simulink model "regtemppid"  (R2025a)
settings: Solver=ode45  StartTime=0.0  StopTime=160000  FixedStep=0.1  RelTol=1e-3  EnableMultiTasking=on
PreLoadFcn:
  | variables;
InitFcn:
  | variables;
values from neighbouring files (symbols this model uses):
  demi_serie = 'A'    [variables.m]
  Kp = 1.05    [variables.m]
  serie = 6    [variables.m]
  set_up = 1    [variables.m]
  T1p = 139.41    [variables.m]
  T2p = 14.29    [variables.m]
  thetap = 9.07    [variables.m]
  Ts = 1    [variables.m]
libraries: simulink x1
settings Model: PacingRate=20  ExtModeTrigMode=oneshot  ExtModeArmWhenConnect=off  Creator=auto2  LastModifiedBy=sabir
settings SolverCC: AlgebraicLoopSolver=TrustRegion
settings DataIOCC: SaveFormat=Array  SignalLoggingSaveFormat=ModelDataLogs  SaveOutput=off  SaveTime=off  ReturnWorkspaceOutputs=off  SignalLoggingName=sigsOut
settings OptimizationCC: BooleanDataType=off  ExpressionDepthLimit=2147483647.0  InitFltsAndDblsToZero=on  LifeSpan=inf
settings DebuggingCC: SaveWithParameterizedLinksMsg=none  UnderspecifiedInitializationDetection=Classic  MergeDetectMultiDrivingBlocksExec=none  SignalResolutionControl=TryResolveAllWithWarning  MultiTaskDSMMsg=warning  MultiTaskCondExecSysMsg=none  FcnCallInpInsideContextMsg=warning  UnconnectedInputMsg=warning  UnconnectedOutputMsg=warning  UnconnectedLineMsg=warning  StateNameClashWarn=warning  SFUnexpectedBacktrackingDiag=warning  SFNoUnconditionalDefaultTransitionDiag=warning  SFExecutionAtInitializationDiag=none  ArithmeticOperatorsInVariantConditions=warning
settings HardwareCC: ProdBitPerPointer=32.0  ProdBitPerSizeT=32.0  ProdBitPerPtrDiffT=32.0  ProdLargestAtomicFloat=None  ProdIntDivRoundTo=Undefined  ProdEndianess=Unspecified  ProdWordSize=32.0  ProdHWDeviceType=32-bit Generic  TargetUnknown=on
settings ModelReferenceCC: EnableRefExpFcnMdlSchedulingChecks=on  PropagateSignalLabelsOutOfModel=off
settings SFSimCC: SimUseLocalCustomCode=off  CustomCodeUndefinedFunction=UseInterfaceOnly
settings RTWCC: RTWUseLocalCustomCode=off  GPUComputeCapability=3.5
settings CodeAppCC: StateflowObjectComments=on
settings GRTTargetCC: TargetLangStandard=C89/C90 (ANSI)  CombineOutputUpdateFcns=off  GRTInterface=on
settings ConfigComp: CovMetricSettings=dw  CovSaveCumulativeToWorkspaceVar=on  CovSaveSingleToWorkspaceVar=on  CovExternalEMLEnable=off  CovSFcnEnable=off

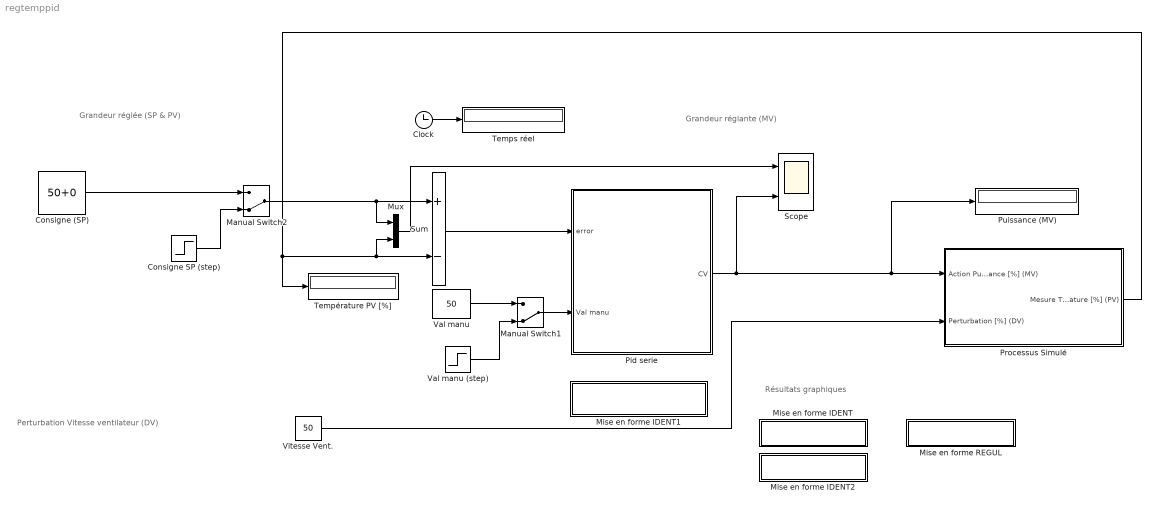
== system regtemppid ==
  note: Grandeur réglante (MV)
  note: Grandeur réglée (SP & PV)
  note: Perturbation Vitesse ventilateur (DV)
  note: Résultats graphiques
  Clock : Clock
      settings: StartFcn=simu(1).bloc_clock='labo'
  Consigne (SP) : Constant  StartFcn=simu(1,1).bloc_SP='labo'  Value=50+0
  Consigne SP (step) : Step  StartFcn=simu(1).bloc_Step_SP='labo'  Time=700  Before=45  After=55  SampleTime=0
  Manual Switch1 : ManualSwitch  CurrentSetting=0
  Manual Switch2 : ManualSwitch  CurrentSetting=0
  Mise en forme IDENT : Subsystem
      settings: OpenFcn=|
      | t=Scope_PID.time;A=[Scope_PID.signals.values];
      | y=A(:,2);u=A(:,3);
      | subplot(211)
      | plot(t,u,'black');
      | title('MV [%]')
      | subplot(212)
      | plot(t,y,'black');
      | title('PV [%]')
      | grid;figure(gcf)
      | 
      | 
      | 
      | tstep=find(diff(u)~=0);
      | tstep=tstep(end); % take last change
      | 
      | tm=t(tstep:end);
      | tm=tm-t(tstep);
      | um=u(tstep:end);
      | um=um-um(1);
      | ym=y(tstep:end);
      | ym=ym-ym(1);
      | 
      | y0 = y(tstep);
      | du = u(end)-u(tstep);
      mask Display: disp('Mise en forme IDENT')
  Mise en forme IDENT1 : Subsystem
      settings: OpenFcn=|
      | string_PID = get_param(bdroot, 'Name');
      | 
      | AMbit=3-length(get_param([string_PID '/Pid serie'],'AMbit'));
      | 
      | if AMbit==1,
      | set_param([string_PID '/Pid serie'],'AMbit','off');
      | AMbit=0;
      | elseif AMbit==0,
      | set_param([string_PID '/Pid serie'],'AMbit','on');
      | AMbit=1;
      | end
      | 
      | 
      | if AMbit==1,
      | 	set_param([string_PID '/Pid serie'],'BackgroundColor','red');
      | 	set_param([string_PID '/Pid serie'],'MaskDisplay','disp(''  PID \n [AUTO]'')');
      | end
      | if AMbit==0,
      | 	set_param([string_PID '/Pid serie'],'BackgroundColor','lightblue');
      | 	set_param([string_PID '/Pid serie'],'MaskDisplay','disp(''  PID \n [MANU]'')');
      | end
      mask Display: disp('Manu <->Auto')
  Mise en forme IDENT2 : Subsystem
      settings: OpenFcn=idoptregtemppidvdg;
      mask Display: disp('IDENT OPT VDG')
  Mise en forme REGUL : Subsystem
      settings: OpenFcn=|
      | t=Scope_PID.time;
      | A=[Scope_PID.signals.values];
      | ysp=A(:,1);
      | u=A(:,3);
      | y=A(:,2);
      | index=min(find(diff(ysp)))-99;
      | subplot(211);
      | y=y(index:end);
      | ysp=ysp(index:end);
      | t=t(index:end);
      | u=u(index:end);
      | plot(t,y,'black',t,ysp,'black');
      | grid;
      | title('PV [%] et SP [%]');
      | subplot(212),
      | plot(t,u,'black');
      | grid;
      | figure(gcf);
      | title('MV [%]')
      mask Display: disp('Mise en forme REGUL');
  Mux : Mux  Inputs=2
  Pid serie : Subsystem  StartFcn=simu(1).bloc_PID='labo'  mask{k=4.82, ti=168, td=10, tf=1, X0=50, lh=100, ll=0, AMbit=on}
      mask prompts: k "Gain"; ti "Temps d'intégration"; td "Temps de dérivation"; tf "Temps de filtrage"; X0 "Valeur initiale de la sortie"; lh "Limite Haute"; ll "Limite basse"; AMbit "Auto [v] / Manu [ ]"
      mask init:
      | string_PID = get_param(bdroot, 'Name');
      | 
      | AMbit=3-length(get_param([string_PID '/Pid serie'],'AMbit'));
      | if AMbit==1,
      | 	set_param([string_PID '/Pid serie'],'BackgroundColor','red');
      | 	set_param([string_PID '/Pid serie'],'MaskDisplay','disp(''  PID \n [AUTO]'')');
      | end
      | if AMbit==0, 
      | 	set_param([string_PID '/Pid serie'],'BackgroundColor','lightblue');
      | 	set_param([string_PID '/Pid serie'],'MaskDisplay','disp(''  PID \n [MANU]'')');
      | end
      mask Display: disp('  PID \n [AUTO]')
  Processus Simulé : Subsystem  StartFcn=simu(1).bloc_Process='labo'  mask{set_up=set_up, serie=serie, demi_serie=demi_serie}
      mask prompts: serie "Série"; demi_serie "Demi série"
      mask init:
      | %%%%%%%%%%%%%%%%%%%%%%%%%%%%%%%%%
      | 
      | switch set_up
      |    case 1
      |         Kd = -0.64;
      |         T1d = 81.54;
      |         T2d = 18.9;
      |         thetad = 12.49;
      |    case 2
      |         Kd = -0.43;
      |         T1d = 34.66;
      |         T2d = 1.13;
      |         thetad = 6.08; 
      |     case 3
      |         Kd = -0.34;
      |         T1d = 82.52;
      |         T2d = 20.99;
      |         thetad = 8.42;  
      | end
      | 
      | if (demi_serie == 'A')
      |     dserie = 1;
      | else
      |     dserie = 5;
      | end    
      | 
      | seed = str2num([num2str(serie) num2str(serie) num2str(dserie) num2str(set_up)]);
      | 
      | rng(seed)
      | x1 = (rand - 1)/5;
      | rng(seed+1)
      | x2 = (rand - 1)/5;
      | rng(seed+2)
      | x3 = (rand - 1)/5;
      | rng(seed+3)
      | x4 = (rand - 1)/5;
      | 
      | Kd = Kd*(1+x1);
      | T1d = T1d*(1+x2);
      | T2d = T2d*(1+x3);
      | thetad =thetad*(1+x4);
  Puissance (MV) : Display
      settings: StartFcn=simu(1).bloc_display_MV='labo'
  Scope : Scope  NumInputPorts=2
      settings: StartFcn=simu(1).bloc_display_scope='labo'  SampleTime=Ts  TimeSpan=1600  Title=SP [%] et PV [%]  ActiveDisplayYMinimum=-7.94952  ActiveDisplayYMaximum=71.54565  DataLoggingMaxPoints=25000  DataLoggingVariableName=Scope_PID
  Sum : Sum  Inputs=+-  InputSameDT=on  SaturateOnIntegerOverflow=on  OutDataTypeStr=Inherit: Same as first input
  Temps réel : Display
      settings: StartFcn=simu(1).bloc_display_clock='labo'
  Température PV [%] : Display
      settings: StartFcn=simu(1).bloc_Display_PV='labo'
  Val manu : Constant  StartFcn=simu(1).bloc_MV='labo'  Value=50
  Val manu (step) : Step  StartFcn=simu(1).bloc_Step_MV='labo'  Time=700  Before=50  After=60  SampleTime=0
  Vitesse Vent. : Constant  StartFcn=simu(1).bloc_DV='labo'  Value=50
  wires:
  Processus Simulé/1(Mesure Température [%] (PV)) -> Température PV [%]/1, Sum/2, Mux/2
  Manual Switch2/1 -> Sum/1, Mux/1
  Sum/1 -> Pid serie/1(error)
  Pid serie/1(CV) -> Processus Simulé/1(Action Puissance [%] (MV)), Puissance (MV)/1, Scope/2
  Vitesse Vent./1 -> Processus Simulé/2(Perturbation [%] (DV))
  Mux/1 -> Scope/1
  Clock/1 -> Temps réel/1
  Val manu (step)/1 -> Manual Switch1/2
  Val manu/1 -> Manual Switch1/1
  Manual Switch1/1 -> Pid serie/2(Val manu)
  Consigne SP (step)/1 -> Manual Switch2/2
  Consigne (SP)/1 -> Manual Switch2/1

== system regtemppid/Mise en forme IDENT ==

== system regtemppid/Mise en forme IDENT1 ==

== system regtemppid/Mise en forme IDENT2 ==

== system regtemppid/Mise en forme REGUL ==

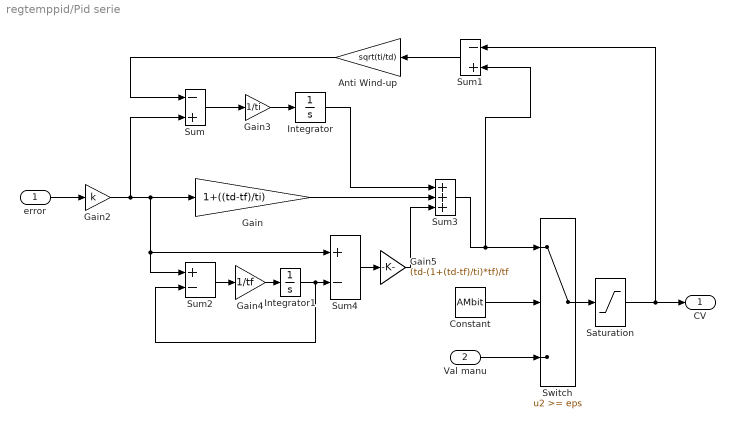
== system regtemppid/Pid serie ==
  error : Inport
  Val manu : Inport  Port=2
  Anti Wind-up : Gain  Gain=sqrt(ti/td)  SaturateOnIntegerOverflow=on  OutDataTypeStr=Inherit: Same as input  ParamDataTypeStr=Inherit: Same as input
  Constant : Constant  Value=AMbit
  Gain : Gain  Gain=1+((td-tf)/ti)  SaturateOnIntegerOverflow=on  OutDataTypeStr=Inherit: Same as input  ParamDataTypeStr=Inherit: Same as input
  Gain2 : Gain  Gain=k  SaturateOnIntegerOverflow=on  OutDataTypeStr=Inherit: Same as input  ParamDataTypeStr=Inherit: Same as input
  Gain3 : Gain  Gain=1/ti  SaturateOnIntegerOverflow=on  OutDataTypeStr=Inherit: Same as input  ParamDataTypeStr=Inherit: Same as input
  Gain4 : Gain  Gain=1/tf  SaturateOnIntegerOverflow=on  OutDataTypeStr=Inherit: Same as input  ParamDataTypeStr=Inherit: Same as input
  Gain5 : Gain  Gain=(td-(1+(td-tf)/ti)*tf)/tf  SaturateOnIntegerOverflow=on  OutDataTypeStr=Inherit: Same as input  ParamDataTypeStr=Inherit: Same as input
  Integrator : Integrator  InitialCondition=X0
  Integrator1 : Integrator
  Saturation : Saturate  UpperLimit=lh  LowerLimit=ll
  Sum : Sum  Inputs=-+  InputSameDT=on  SaturateOnIntegerOverflow=on  OutDataTypeStr=Inherit: Same as first input
  Sum1 : Sum  Inputs=-+  InputSameDT=on  SaturateOnIntegerOverflow=on  OutDataTypeStr=Inherit: Same as first input
  Sum2 : Sum  Inputs=+-  InputSameDT=on  SaturateOnIntegerOverflow=on  OutDataTypeStr=Inherit: Same as first input
  Sum3 : Sum  Inputs=+++  InputSameDT=on  SaturateOnIntegerOverflow=on  OutDataTypeStr=Inherit: Same as first input
  Sum4 : Sum  Inputs=+-  InputSameDT=on  SaturateOnIntegerOverflow=on  OutDataTypeStr=Inherit: Same as first input
  Switch : Switch  Threshold=eps
  CV : Outport
  wires:
  Saturation/1 -> Sum1/1, CV/1
  Switch/1 -> Saturation/1
  Val manu/1 -> Switch/3
  Constant/1 -> Switch/2
  error/1 -> Gain2/1
  Sum1/1 -> Anti Wind-up/1
  Anti Wind-up/1 -> Sum/1
  Sum3/1 -> Switch/1, Sum1/2
  Sum/1 -> Gain3/1
  Gain2/1 -> Sum/2, Gain/1, Sum2/1, Sum4/1
  Gain/1 -> Sum3/2
  Gain3/1 -> Integrator/1
  Integrator/1 -> Sum3/1
  Sum2/1 -> Gain4/1
  Gain4/1 -> Integrator1/1
  Sum4/1 -> Gain5/1
  Integrator1/1 -> Sum4/2, Sum2/2
  Gain5/1 -> Sum3/3

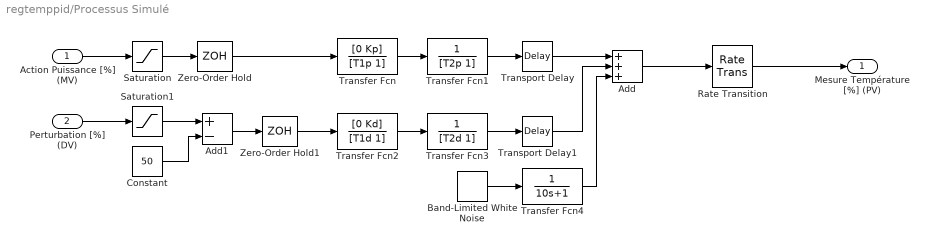
== system regtemppid/Processus Simulé ==
  Action Puissance [%] (MV) : Inport
  Perturbation [%] (DV) : Inport  Port=2
  Add : Sum  Inputs=+++
  Add1 : Sum  Inputs=+-
  Band-Limited White Noise : simulink/Sources/Band-Limited White Noise  Cov=[0.1]  Ts=Ts  seed=[23341]
  Constant : Constant  Value=50  SampleTime=Inf
  Rate Transition : RateTransition  OutPortSampleTime=Ts
  Saturation : Saturate  UpperLimit=100  LowerLimit=0
  Saturation1 : Saturate  UpperLimit=100  LowerLimit=0
  Transfer Fcn : TransferFcn  Numerator=[0 Kp]  Denominator=[T1p 1]
  Transfer Fcn1 : TransferFcn  Numerator=[0 1]  Denominator=[T2p 1]
  Transfer Fcn2 : TransferFcn  Numerator=[0 Kd]  Denominator=[T1d 1]
  Transfer Fcn3 : TransferFcn  Numerator=[0 1]  Denominator=[T2d 1]
  Transfer Fcn4 : TransferFcn  Numerator=[0 1]  Denominator=[10 1]
  Transport Delay : TransportDelay  DelayTime=thetap
  Transport Delay1 : TransportDelay  DelayTime=thetad
  Zero-Order Hold : ZeroOrderHold  SampleTime=Ts
  Zero-Order Hold1 : ZeroOrderHold  SampleTime=Ts
  Mesure Température [%] (PV) : Outport
  wires:
  Transfer Fcn/1 -> Transfer Fcn1/1
  Transfer Fcn1/1 -> Transport Delay/1
  Transport Delay/1 -> Add/1
  Constant/1 -> Add1/2
  Transfer Fcn2/1 -> Transfer Fcn3/1
  Transfer Fcn3/1 -> Transport Delay1/1
  Add1/1 -> Zero-Order Hold1/1
  Add/1 -> Rate Transition/1
  Zero-Order Hold/1 -> Transfer Fcn/1
  Saturation1/1 -> Add1/1
  Saturation/1 -> Zero-Order Hold/1
  Transport Delay1/1 -> Add/2
  Zero-Order Hold1/1 -> Transfer Fcn2/1
  Action Puissance [%] (MV)/1 -> Saturation/1
  Perturbation [%] (DV)/1 -> Saturation1/1
  Rate Transition/1 -> Mesure Température [%] (PV)/1
  Band-Limited White Noise/1 -> Transfer Fcn4/1
  Transfer Fcn4/1 -> Add/3
